simulink model "OneCombinedLQR"  (R2025b)
settings: Solver=ode4  StartTime=0.0  StopTime=T_end  FixedStep=0.005  RelTol=1e-3
values from neighbouring files (symbols this model uses):
  K_lqr = double(K_lqr)    [main.m]
  P = [x_ref y_ref]    [main.m]
  S_path = [S_path; S_raw(end)]    [main.m]
  theta_ref_unwrapped = unwrap(theta_ref)    [main.m]
  vd_path = min(vd_path, vd_max)    [main.m]
  wd_path = max(min(wd_path, wd_max), -wd_max)    [main.m]
settings Model: Creator=mwali  LastModifiedBy=mwali

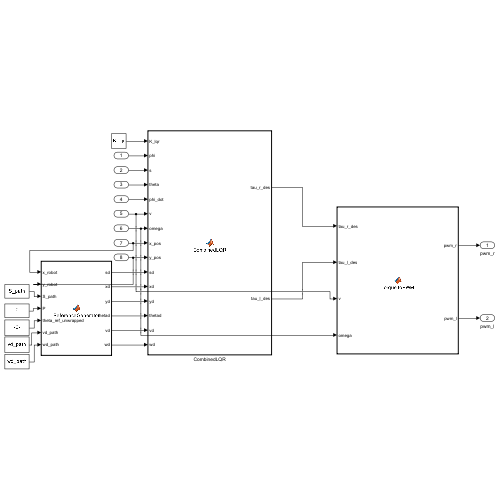
[thumbnail: Simulink's stored preview of the top-level diagram]
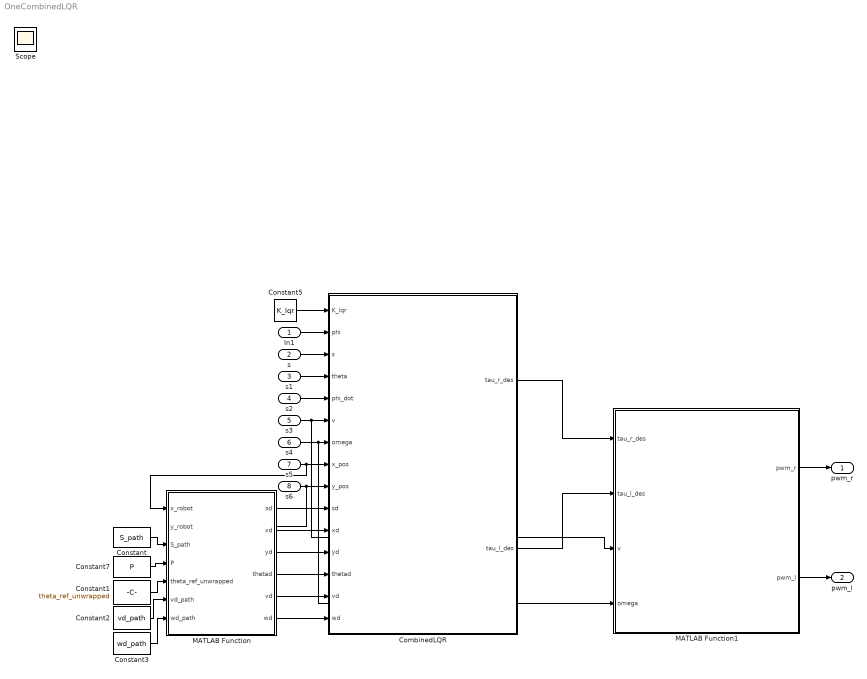
== system OneCombinedLQR ==
  In1 : Inport
  s : Inport  Port=2
  s1 : Inport  Port=3
  s2 : Inport  Port=4
  s3 : Inport  Port=5
  s4 : Inport  Port=6
  s5 : Inport  Port=7
  s6 : Inport  Port=8
  CombinedLQR : MATLAB Function  TreatAsAtomicUnit=on
  Constant : Constant  Value=S_path
  Constant1 : Constant  Value=theta_ref_unwrapped
  Constant2 : Constant  Value=vd_path
  Constant3 : Constant  Value=wd_path
  Constant5 : Constant  Value=K_lqr
  Constant7 : Constant  Value=P
  MATLAB Function : MATLAB Function  TreatAsAtomicUnit=on
  MATLAB Function1 : MATLAB Function  TreatAsAtomicUnit=on
  pwm_r : Outport
  pwm_l : Outport  Port=2
  Scope : Scope
      settings: ActiveDisplayYMinimum=-0.34848844243079913  ActiveDisplayYMaximum=2.6945477005962535
  wires:
  MATLAB Function/2(xd) -> CombinedLQR/11(xd)
  s2/1 -> CombinedLQR/5(phi_dot)
  s1/1 -> CombinedLQR/4(theta)
  Constant1/1 -> MATLAB Function/5(theta_ref_unwrapped)
  Constant/1 -> MATLAB Function/3(S_path)
  Constant3/1 -> MATLAB Function/7(wd_path)
  MATLAB Function/3(yd) -> CombinedLQR/12(yd)
  s6/1 -> MATLAB Function/2(y_robot), CombinedLQR/9(y_pos)
  s3/1 -> MATLAB Function1/3(v), CombinedLQR/6(v)
  s4/1 -> MATLAB Function1/4(omega), CombinedLQR/7(omega)
  s5/1 -> MATLAB Function/1(x_robot), CombinedLQR/8(x_pos)
  s/1 -> CombinedLQR/3(s)
  Constant2/1 -> MATLAB Function/6(vd_path)
  MATLAB Function1/2(pwm_l) -> pwm_l/1
  MATLAB Function1/1(pwm_r) -> pwm_r/1
  MATLAB Function/1(sd) -> CombinedLQR/10(sd)
  Constant7/1 -> MATLAB Function/4(P)
  CombinedLQR/1(tau_r_des) -> MATLAB Function1/1(tau_r_des)
  CombinedLQR/2(tau_l_des) -> MATLAB Function1/2(tau_l_des)
  MATLAB Function/6(wd) -> CombinedLQR/15(wd)
  MATLAB Function/4(thetad) -> CombinedLQR/13(thetad)
  In1/1 -> CombinedLQR/2(phi)
  MATLAB Function/5(vd) -> CombinedLQR/14(vd)
  Constant5/1 -> CombinedLQR/1(K_lqr)

== matlab function OneCombinedLQR/CombinedLQR ==
  settings: updateMethod=DISCRETE
  data: K_lqr input; phi input; s input; theta input; phi_dot input; v input; omega input; x_pos input; y_pos input; sd input; xd input; yd input; thetad input; vd input; wd input; tau_r_des output; tau_l_des output
function [tau_r_des, tau_l_des] = CombinedLQR( ...
    K_lqr, phi, s, theta, phi_dot, v, omega, x_pos, y_pos, ...
    sd, xd, yd, thetad, vd, wd)
%#codegen

% outputs init
tau_r_des  = 0;
tau_l_des  = 0;
ex_out     = 0;
ey_out     = 0;
etheta_out = 0;

% -----------------------------
% 1) Path position error in world frame
% -----------------------------
dx = xd - x_pos;
dy = yd - y_pos;

% -----------------------------
% 2) Error in robot body frame
% ex = forward error
% et = lateral error
% -----------------------------
ex =  cos(theta)*dx + sin(theta)*dy;
ey = -sin(theta)*dx + cos(theta)*dy;

% save for plotting
ex_out = ex;
ey_out = ey;

% -----------------------------
% 3) Heading correction from lateral error
% -----------------------------
k_y = 0.1;                     % tune this if needed
theta_corr_max = deg2rad(20);  % max heading correction

theta_corr = k_y * ey;

if theta_corr > theta_corr_max
    theta_corr = theta_corr_max;
elseif theta_corr < -theta_corr_max
    theta_corr = -theta_corr_max;
end

thetad_corr = thetad + theta_corr;

% -----------------------------
% 4) State error for LQR
% -----------------------------
e = zeros(6,1);
e(1) =phi ;
e(2) = s - sd; 
e(3) = atan2(sin(theta - thetad_corr), cos(theta - thetad_corr));
e(4) = phi_dot;
e(5) = v - vd;
e(6) = omega - wd;

etheta_out = e(3);

% -----------------------------
% 5) LQR control
% -----------------------------
u_des = -K_lqr * e;

tau_r_des = u_des(1);
tau_l_des = u_des(2);

% -----------------------------
% 6) Torque saturation
% -----------------------------
tau_lim = 3; % Changed from 6 to 3

if tau_r_des > tau_lim
    tau_r_des = tau_lim;
elseif tau_r_des < -tau_lim
    tau_r_des = -tau_lim;
end

if tau_l_des > tau_lim
    tau_l_des = tau_lim;
elseif tau_l_des < -tau_lim
    tau_l_des = -tau_lim;
end

== matlab function OneCombinedLQR/MATLAB Function ==
  data: x_robot input; y_robot input; S_path input; P input; theta_ref_unwrapped input; vd_path input; wd_path input; sd output; xd output; yd output; thetad output; vd output; wd output
function [sd, xd, yd, thetad, vd, wd] = ReferenceGenerator(x_robot, y_robot, S_path, P, theta_ref_unwrapped, vd_path, wd_path)
    N = size(P, 1);

    % 1. Find the nearest discrete node
    min_dist2 = inf;
    k_min = int32(1);
    for k = int32(1) : int32(N)
        dx = P(k, 1) - x_robot;
        dy = P(k, 2) - y_robot;
        d2 = dx*dx + dy*dy;
        if d2 < min_dist2
            min_dist2 = d2;
            k_min = k;
        end
    end

    % 2. Continuous Projection (Fixes the high-frequency torque chattering)
    k_next = min(k_min + int32(1), int32(N));
    k_prev = max(k_min - int32(1), int32(1));

    d2_next = (P(k_next,1)-x_robot)^2 + (P(k_next,2)-y_robot)^2;
    d2_prev = (P(k_prev,1)-x_robot)^2 + (P(k_prev,2)-y_robot)^2;

    if d2_next < d2_prev
        k1 = k_min;
        k2 = k_next;
    else
        k1 = k_prev;
        k2 = k_min;
    end

    if k1 == k2
        alpha = 0.0;
    else
        vx = P(k2,1) - P(k1,1);
        vy = P(k2,2) - P(k1,2);
        L2 = vx*vx + vy*vy;
        if L2 > 1e-6
            rx = x_robot - P(k1,1);
            ry = y_robot - P(k1,2);
            % Orthogonal projection scalar
            alpha = (rx*vx + ry*vy) / L2;
            alpha = max(0.0, min(1.0, alpha));
        else
            alpha = 0.0;
        end
    end

    % 3. Interpolate perfectly smooth references (No Lookahead)
    sd     = (1 - alpha) * S_path(k1) + alpha * S_path(k2);
    xd     = (1 - alpha) * P(k1, 1)   + alpha * P(k2, 1);
    yd     = (1 - alpha) * P(k1, 2)   + alpha * P(k2, 2);
    thetad = (1 - alpha) * theta_ref_unwrapped(k1) + alpha * theta_ref_unwrapped(k2);
    vd     = (1 - alpha) * vd_path(k1) + alpha * vd_path(k2);
    wd     = (1 - alpha) * wd_path(k1) + alpha * wd_path(k2);

    % 4. Safety clamps
    vd_max = 0.3;
    wd_max = 0.334;
    vd = max(0, min(vd, vd_max));
    wd = max(min(wd, wd_max), -wd_max);
end

== matlab function OneCombinedLQR/MATLAB Function1 ==
  data: tau_r_des input; pwm_r output; tau_l_des input; v input; omega input; pwm_l output
function [pwm_r, pwm_l] = TorqueToPWM(tau_r_des, tau_l_des, v, omega)
    % --- NFP-42GP-775-EN Motor Parameters ---
    K_t = 0.6746;      % Torque constant (Nm/A)
    K_e = 0.6746;      % Back-EMF constant (V/(rad/s))
    R_res = 0.9796;    % Armature resistance (Ohms)
    V_batt = 24.0;     % Battery voltage (V)
    
    % --- Controller & Robot Parameters ---
    max_pwm = 255;     % Change this if using a 10-bit or 12-bit timer!
    r = 0.060;         % Wheel radius (m)
    d = 0.450;         % Wheelbase/Track width (m)

    % 1. Estimate individual wheel rotational speeds (rad/s)
    omega_wheel_r = (v + (omega * d / 2)) / r;
    omega_wheel_l = (v - (omega * d / 2)) / r;

    % 2. Calculate right wheel PWM
    i_r = tau_r_des / K_t;
    v_r = (i_r * R_res) + (K_e * omega_wheel_r);
    pwm_float_r = (v_r / V_batt) * max_pwm;

    % 3. Calculate left wheel PWM
    i_l = tau_l_des / K_t;
    v_l = (i_l * R_res) + (K_e * omega_wheel_l);
    pwm_float_l = (v_l / V_batt) * max_pwm;

    % 4. Round to integer and clamp to valid ranges
    pwm_r = round(pwm_float_r);
    pwm_l = round(pwm_float_l);

    if pwm_r > max_pwm
        pwm_r = max_pwm; 
    elseif pwm_r < -max_pwm
        pwm_r = -max_pwm; 
    end
    
    if pwm_l > max_pwm
        pwm_l = max_pwm; 
    elseif pwm_l < -max_pwm
        pwm_l = -max_pwm; 
    end
end
